simulink model "Prova_SS"  (R2022b)
settings: Solver=VariableStepAuto  StartTime=0.0  StopTime=10.0  RelTol=1e-3
values from neighbouring files (symbols this model uses):
  Nu = X(3)    [Prova_es2.m]    (also in Prova_es2_MIK.m)
  Nx = X(1:2)    [Prova_es2.m]    (also in Prova_es2_MIK.m)
undefined symbols (not defined in the file or in its folder): degs2rpm, Ke, Kw, nom, rpm2rads, sens
settings Model: Creator=marcoverri  LastModifiedBy=marcoverri

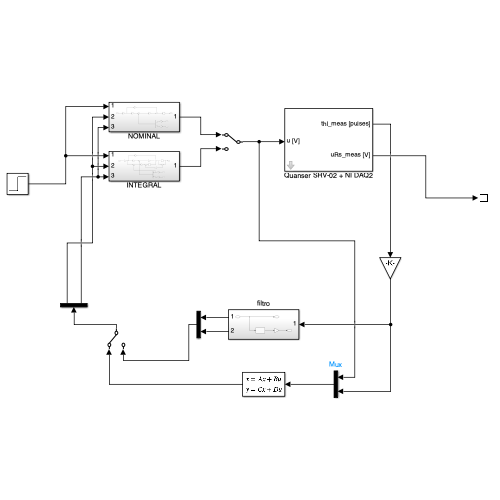
[thumbnail: Simulink's stored preview of the top-level diagram]
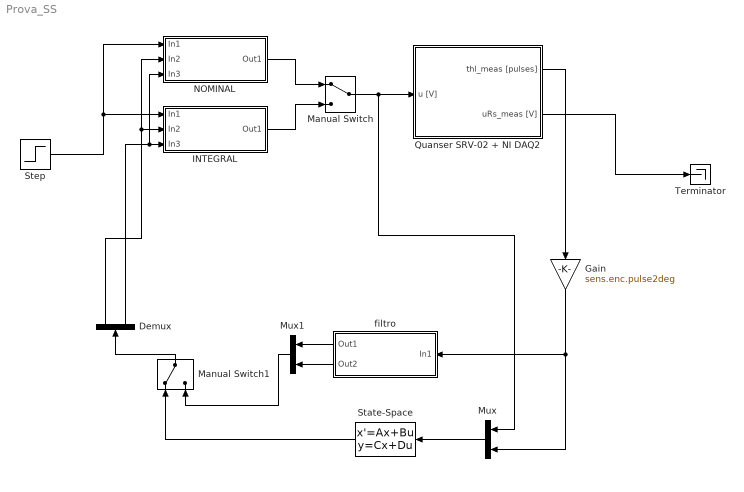
== system Prova_SS ==
  Demux : Demux  Outputs=2
  Gain : Gain  Gain=sens.enc.pulse2deg
  INTEGRAL : Subsystem
  Manual Switch : ManualSwitch
  Manual Switch1 : ManualSwitch
  Mux : Mux  Inputs=2
  Mux1 : Mux  Inputs=2
  NOMINAL : Subsystem
  Quanser SRV-02 + NI DAQ2 : Subsystem  mask(Quanser SRV-02 (with inertial load) + NI DAQ){Ts=0.001, fricType=Coulomb + viscous}
      mask prompts: Ts "NI DAQ Sample Time:"; fricType "Friction model"
      mask help: Quanser SRV-02 (with inertial load) + NI DAQ model.
      mask init:
      | %%  Sensors data
      | 
      | %   shunt resistor
      | sens.curr.Rs = 0.5;                         %   resistance [Ohm]   
      | sens.curr.uRs_std = 0.01;                   %   voltage noise standard dev [V]                           
      | sens.curr.uRs_var = sens.curr.uRs_std^2;	%   voltage noise variance [V^2]
      | 
      | %   Hewlett-Packard HEDS-5540#A06 optical encoder
      | sens.enc.ppr = 500*4;                       %   pulses per rotation
      | sens.enc.pulse2deg = 360/sens.enc.ppr;      %   [pulses] -> [deg]
      | sens.enc.pulse2rad = 2*pi/sens.enc.ppr;     %   [pulses] -> [rad]
      | sens.enc.deg2pulse = sens.enc.ppr/360;      %   [deg] -> [pulses]
      | sens.enc.rad2pulse = sens.enc.ppr/2/pi;     %   [rad] -> [pulses]
      | 
      | 
      | %%  Data acquisition board (daq) data
      | 
      | %   NI PCI-6221 DAC data
      | daq.dac.bits = 16;                                  %   resolution (bits)
      | daq.dac.fs   = 10;                                  %   full scale 
      | daq.dac.q    = 2*daq.dac.fs/(2^daq.dac.bits-1);     %	quantization
      | 
      | %   NI PCI-6221 ADC data
      | daq.adc.bits = 16;                                  %   resolution (bits)
      | daq.adc.fs   = 10;                                  %   full scale (as set in SLDRT Analog Input block)
      | daq.adc.q    = 2*daq.adc.fs/(2^daq.adc.bits-1);     %   quantization
      mask Help:
      | Riccardo Antonello (antonello@dei.unipd.it)
      | 
      | April 24, 2020
      | 
      | Dept. of Information Engineering, University of Padova
      mask TypeOptions fricType: Coulomb + viscous | Karnopp
  State-Space : StateSpace  InitialCondition=0
  Step : Step  SampleTime=0
  Terminator : Terminator
  filtro : Subsystem
  wires:
  Step/1 -> INTEGRAL/1(In1), NOMINAL/1(In1)
  Quanser SRV-02 + NI DAQ2/2(uRs_meas [V]) -> Terminator/1
  Quanser SRV-02 + NI DAQ2/1(thl_meas [pulses]) -> Gain/1
  Gain/1 -> Mux/2, filtro/1(In1)
  NOMINAL/1(Out1) -> Manual Switch/1
  INTEGRAL/1(Out1) -> Manual Switch/2
  State-Space/1 -> Manual Switch1/1
  Mux/1 -> State-Space/1
  Manual Switch/1 -> Mux/1, Quanser SRV-02 + NI DAQ2/1(u [V])
  filtro/1(Out1) -> Mux1/1
  filtro/2(Out2) -> Mux1/2
  Mux1/1 -> Manual Switch1/2
  Manual Switch1/1 -> Demux/1
  Demux/1 -> NOMINAL/2(In2), INTEGRAL/2(In2)
  Demux/2 -> INTEGRAL/3(In3), NOMINAL/3(In3)

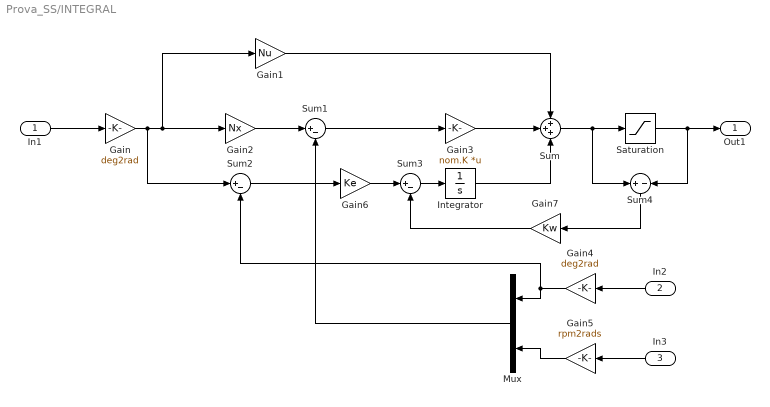
== system Prova_SS/INTEGRAL ==
  In1 : Inport
  In2 : Inport  Port=2
  In3 : Inport  Port=3
  Gain : Gain  Gain=deg2rad
  Gain1 : Gain  Gain=Nu
  Gain2 : Gain  Gain=Nx
  Gain3 : Gain  Gain=nom.K  Multiplication=Matrix(K*u)
  Gain4 : Gain  Gain=deg2rad
  Gain5 : Gain  Gain=rpm2rads
  Gain6 : Gain  Gain=Ke
  Gain7 : Gain  Gain=Kw
  Integrator : Integrator
  Mux : Mux  Inputs=2
  Saturation : Saturate  UpperLimit=10  LowerLimit=-10
  Sum : Sum  Inputs=+++
  Sum1 : Sum  Inputs=|+-
  Sum2 : Sum  Inputs=|+-
  Sum3 : Sum  Inputs=|+-
  Sum4 : Sum  Inputs=+-
  Out1 : Outport
  wires:
  In1/1 -> Gain/1
  Gain/1 -> Sum2/1, Gain1/1, Gain2/1
  Gain1/1 -> Sum/1
  Gain3/1 -> Sum/2
  Sum1/1 -> Gain3/1
  Sum/1 -> Sum4/1, Saturation/1
  Saturation/1 -> Sum4/2, Out1/1
  Gain2/1 -> Sum1/1
  In3/1 -> Gain5/1
  In2/1 -> Gain4/1
  Gain4/1 -> Sum2/2, Mux/1
  Gain5/1 -> Mux/2
  Mux/1 -> Sum1/2
  Integrator/1 -> Sum/3
  Sum2/1 -> Gain6/1
  Gain6/1 -> Sum3/1
  Sum3/1 -> Integrator/1
  Sum4/1 -> Gain7/1
  Gain7/1 -> Sum3/2

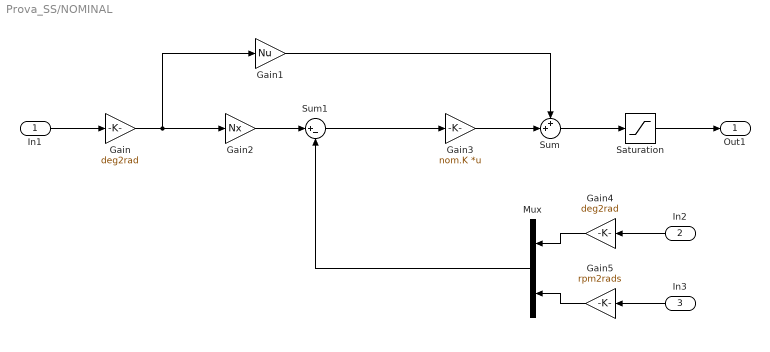
== system Prova_SS/NOMINAL ==
  In1 : Inport
  In2 : Inport  Port=2
  In3 : Inport  Port=3
  Gain : Gain  Gain=deg2rad
  Gain1 : Gain  Gain=Nu
  Gain2 : Gain  Gain=Nx
  Gain3 : Gain  Gain=nom.K  Multiplication=Matrix(K*u)
  Gain4 : Gain  Gain=deg2rad
  Gain5 : Gain  Gain=rpm2rads
  Mux : Mux  Inputs=2
  Saturation : Saturate  UpperLimit=10  LowerLimit=-10
  Sum : Sum  Inputs=++|
  Sum1 : Sum  Inputs=|+-
  Out1 : Outport
  wires:
  In1/1 -> Gain/1
  Gain/1 -> Gain1/1, Gain2/1
  Gain1/1 -> Sum/1
  Gain3/1 -> Sum/2
  Sum1/1 -> Gain3/1
  Sum/1 -> Saturation/1
  Saturation/1 -> Out1/1
  Gain2/1 -> Sum1/1
  In3/1 -> Gain5/1
  In2/1 -> Gain4/1
  Gain4/1 -> Mux/1
  Gain5/1 -> Mux/2
  Mux/1 -> Sum1/2

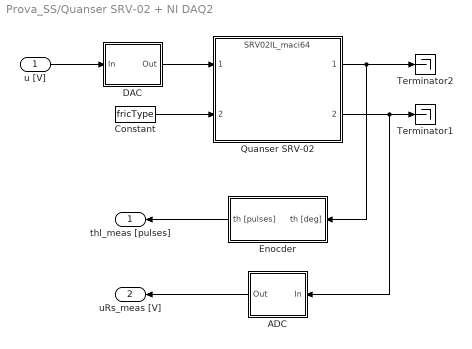
== system Prova_SS/Quanser SRV-02 + NI DAQ2 ==
  u [V] : Inport
  ADC : Subsystem
  Constant : Constant  Value=fricType
  DAC : Subsystem
  Enocder : Subsystem
  Quanser SRV-02 : ModelReference  ModelNameDialog=SRV02IL_maci64.slxp  ModelReferenceVersion=1.44  CopyOfModelProtected=on
  Terminator1 : Terminator
  Terminator2 : Terminator
  thl_meas [pulses] : Outport
  uRs_meas [V] : Outport  Port=2
  wires:
  Enocder/1(th [pulses]) -> thl_meas [pulses]/1
  ADC/1(Out) -> uRs_meas [V]/1
  DAC/1(Out) -> Quanser SRV-02/1
  Quanser SRV-02/2 -> ADC/1(In), Terminator1/1
  u [V]/1 -> DAC/1(In)
  Quanser SRV-02/1 -> Enocder/1(th [deg]), Terminator2/1
  Constant/1 -> Quanser SRV-02/2

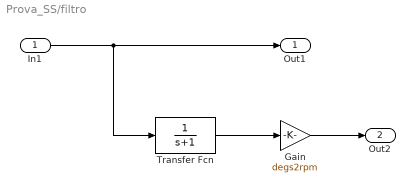
== system Prova_SS/filtro ==
  In1 : Inport
  Gain : Gain  Gain=degs2rpm
  Transfer Fcn : TransferFcn  Denominator=[1 1]
  Out1 : Outport
  Out2 : Outport  Port=2
  wires:
  Transfer Fcn/1 -> Gain/1
  In1/1 -> Transfer Fcn/1, Out1/1
  Gain/1 -> Out2/1

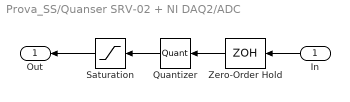
== system Prova_SS/Quanser SRV-02 + NI DAQ2/ADC ==
  In : Inport
  Quantizer : Quantizer  QuantizationInterval=daq.adc.q
  Saturation : Saturate  UpperLimit=daq.adc.fs  LowerLimit=-daq.adc.fs
  Zero-Order Hold : ZeroOrderHold  SampleTime=Ts
  Out : Outport
  wires:
  Saturation/1 -> Out/1
  In/1 -> Zero-Order Hold/1
  Quantizer/1 -> Saturation/1
  Zero-Order Hold/1 -> Quantizer/1

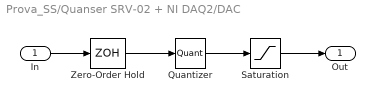
== system Prova_SS/Quanser SRV-02 + NI DAQ2/DAC ==
  In : Inport
  Quantizer : Quantizer  QuantizationInterval=daq.dac.q
  Saturation : Saturate  UpperLimit=daq.dac.fs  LowerLimit=-daq.dac.fs
  Zero-Order Hold : ZeroOrderHold  SampleTime=Ts
  Out : Outport
  wires:
  Quantizer/1 -> Saturation/1
  In/1 -> Zero-Order Hold/1
  Zero-Order Hold/1 -> Quantizer/1
  Saturation/1 -> Out/1

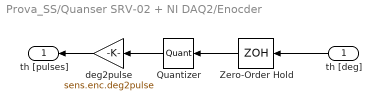
== system Prova_SS/Quanser SRV-02 + NI DAQ2/Enocder ==
  th [deg] : Inport
  Quantizer : Quantizer  QuantizationInterval=sens.enc.pulse2deg
  Zero-Order Hold : ZeroOrderHold  SampleTime=Ts
  deg2pulse : Gain  Gain=sens.enc.deg2pulse
  th [pulses] : Outport
  wires:
  Quantizer/1 -> deg2pulse/1
  th [deg]/1 -> Zero-Order Hold/1
  Zero-Order Hold/1 -> Quantizer/1
  deg2pulse/1 -> th [pulses]/1
